simulink subsystem "MemoryInputDriver"  (R2024b)
settings: Solver=VariableStepAuto  StartTime=0.0  StopTime=10.0  RelTol=1e-3
model mask{absoluteAddress=0, MemoryNWords=0, registerDataType=uint32}
  mask prompts: absoluteAddress "Memory Absolute Address"; MemoryNWords "Memory Size (Words)"; registerDataType "Register Data Type"
undefined symbols (not defined in the file): SimuRISC_Constants
libraries: simulink x3, hdlsllib x1
settings Model: Creator=stefano  LastModifiedBy=stefano

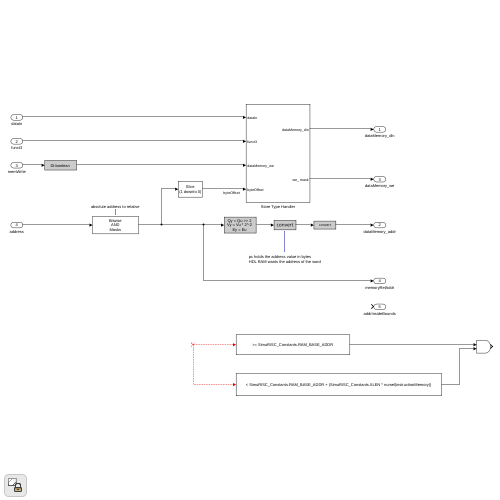
[thumbnail: Simulink's stored preview of the top-level diagram]
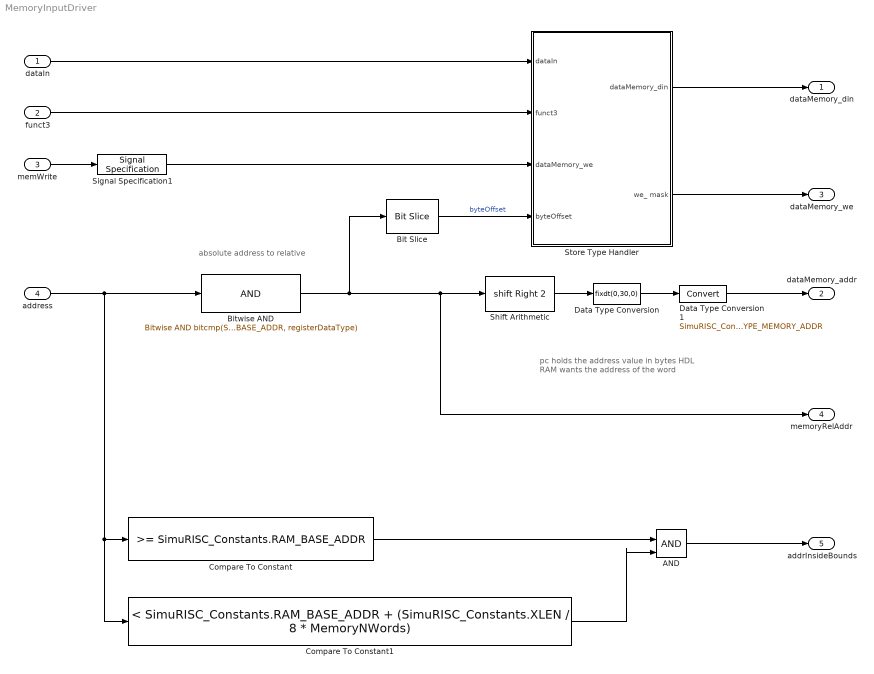
== system MemoryInputDriver ==
  note: pc holds the address value in bytes
      | HDL RAM wants the address of the word
  note: absolute address to relative
  dataIn : Inport
  funct3 : Inport  Port=2
  memWrite : Inport  Port=3
  address : Inport  Port=4
  AND : Logic  IconShape=distinctive  AllPortsSameDT=off  OutDataTypeStr=boolean
  Bit Slice : hdlsllib/Logic and Bit Operations/Bit Slice  lidx=1  ridx=0
  Bitwise AND : simulink/Logic and Bit Operations/Bitwise Operator  logicop=AND  UseBitMask=on  BitMask=bitcmp(SimuRISC_Constants.RAM_BASE_ADDR, registerDataType)  BitMaskRealWorld=Stored Integer
      settings: LibrarySourceBlock=|
      | simulink/Quick Insert/Logic and Bit
      | Operations/Bitwise AND
  Compare To Constant : simulink/Logic and Bit Operations/Compare To Constant  relop=>=  const=SimuRISC_Constants.RAM_BASE_ADDR  OutDataTypeStr=boolean
  Compare To Constant1 : simulink/Logic and Bit Operations/Compare To Constant  relop=<  const=SimuRISC_Constants.RAM_BASE_ADDR + (SimuRISC_Constants.XLEN / 8 * MemoryNWords)  OutDataTypeStr=boolean
  Data Type Conversion : DataTypeConversion  OutDataTypeStr=fixdt(0,30,0)  SaturateOnIntegerOverflow=off  RndMeth=Floor
  Data Type Conversion1 : DataTypeConversion  OutDataTypeStr=SimuRISC_Constants.DATATYPE_MEMORY_ADDR  SaturateOnIntegerOverflow=off  RndMeth=Floor
  Shift Arithmetic : ArithShift  BitShiftNumber=2  BitShiftDirection=Right
  Signal Specification1 : SignalSpecification  OutDataTypeStr=boolean
  Store Type Handler : Subsystem
  dataMemory_din : Outport
  dataMemory_addr : Outport  Port=2
  dataMemory_we : Outport  Port=3
  memoryRelAddr : Outport  Port=4
  addrInsideBounds : Outport  Port=5
  wires:
  Shift Arithmetic/1 -> Data Type Conversion/1
  Data Type Conversion/1 -> Data Type Conversion1/1
  dataIn/1 -> Store Type Handler/1(dataIn)
  funct3/1 -> Store Type Handler/2(funct3)
  Bit Slice/1 -> Store Type Handler/4(byteOffset)  "byteOffset"
  Store Type Handler/1(dataMemory_din) -> dataMemory_din/1
  memWrite/1 -> Signal Specification1/1
  Store Type Handler/2(we_ mask) -> dataMemory_we/1
  Data Type Conversion1/1 -> dataMemory_addr/1
  Signal Specification1/1 -> Store Type Handler/3(dataMemory_we)
  Bitwise AND/1 -> Bit Slice/1, Shift Arithmetic/1, memoryRelAddr/1
  Compare To Constant/1 -> AND/1
  Compare To Constant1/1 -> AND/2
  address/1 -> Bitwise AND/1, Compare To Constant/1, Compare To Constant1/1
  AND/1 -> addrInsideBounds/1

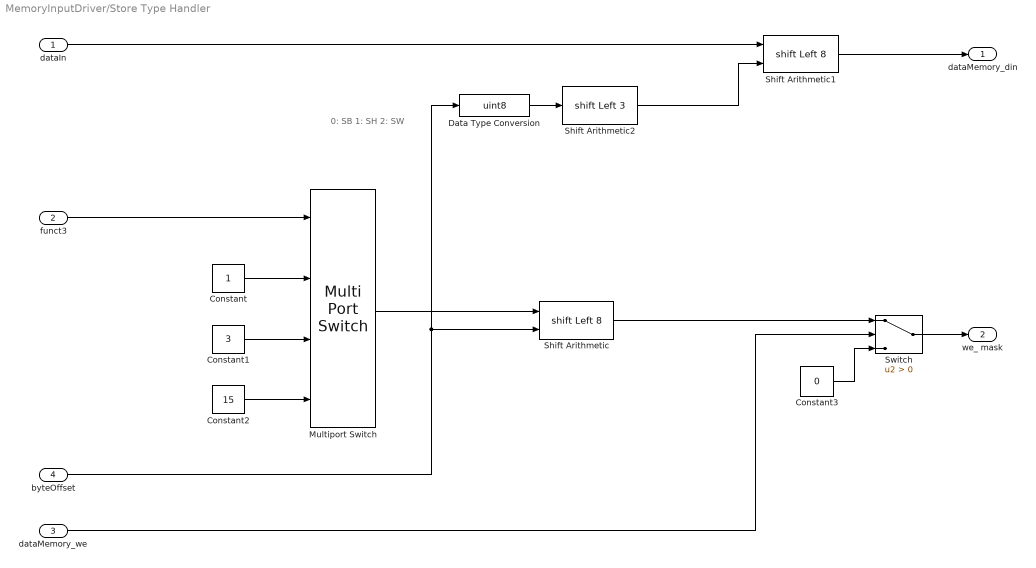
== system MemoryInputDriver/Store Type Handler ==
  note: 0: SB
      | 1: SH
      | 2: SW
  dataIn : Inport
  funct3 : Inport  Port=2
  dataMemory_we : Inport  Port=3
  byteOffset : Inport  Port=4
  Constant : Constant  OutDataTypeStr=fixdt(0,4,0)  SampleTime=-1
  Constant1 : Constant  Value=3  OutDataTypeStr=fixdt(0,4,0)  SampleTime=-1
  Constant2 : Constant  Value=15  OutDataTypeStr=fixdt(0,4,0)  SampleTime=-1
  Constant3 : Constant  Value=0  OutDataTypeStr=fixdt(0,4,0)  SampleTime=-1
  Data Type Conversion : DataTypeConversion  OutDataTypeStr=uint8  SaturateOnIntegerOverflow=off  RndMeth=Floor
  Multiport Switch : MultiPortSwitch  DataPortOrder=Zero-based contiguous  DataPortIndices={0,1,2,4,5}  DiagnosticForDefault=None  zeroidx=on  SaturateOnIntegerOverflow=off  InputSameDT=off
  Shift Arithmetic : ArithShift  BitShiftNumberSource=Input port  BitShiftNumber=8  BitShiftDirection=Left
      settings: InputPortMap=u0,p1
  Shift Arithmetic1 : ArithShift  BitShiftNumberSource=Input port  BitShiftNumber=8  BitShiftDirection=Left
      settings: InputPortMap=u0,p1
  Shift Arithmetic2 : ArithShift  BitShiftNumber=3  BitShiftDirection=Left
  Switch : Switch  Criteria=u2 > Threshold  SaturateOnIntegerOverflow=off  InputSameDT=off
  dataMemory_din : Outport
  we_ mask : Outport  Port=2
  wires:
  Shift Arithmetic2/1 -> Shift Arithmetic1/2
  Data Type Conversion/1 -> Shift Arithmetic2/1
  Shift Arithmetic1/1 -> dataMemory_din/1
  dataIn/1 -> Shift Arithmetic1/1
  Constant3/1 -> Switch/3
  Constant2/1 -> Multiport Switch/4
  Switch/1 -> we_ mask/1
  dataMemory_we/1 -> Switch/2
  byteOffset/1 -> Data Type Conversion/1, Shift Arithmetic/2
  Shift Arithmetic/1 -> Switch/1
  funct3/1 -> Multiport Switch/1
  Constant/1 -> Multiport Switch/2
  Constant1/1 -> Multiport Switch/3
  Multiport Switch/1 -> Shift Arithmetic/1
